simulink model "lab2_teste"  (R2017a)
settings: Solver=ode3  StartTime=0.0  StopTime=10.0  RelTol=1e-3  EnableMultiTasking=on
values from neighbouring files (symbols this model uses):
  input_amplitude = 1    [test2_square_half_hz.mat]
  input_frequency = 0.5    [test2_square_half_hz.mat]
  sampling_time = 0.02    [prbs_good_b0-098.mat]    (also in test2_square_half_hz.mat)
undefined symbols (not defined in the file or in its folder): MIO, National_Instruments, PCI
libraries: sldrtlib x3
settings Model: SimulationMode=external  ExtModeTrigDuration=20000  Creator=alunos  LastModifiedBy=jmgri
settings DataIOCC: SaveFormat=Array
settings DebuggingCC: SFUnexpectedBacktrackingDiag=warning  SFNoUnconditionalDefaultTransitionDiag=warning  SFExecutionAtInitializationDiag=none
settings HardwareCC: TargetIntDivRoundTo=Zero  TargetEndianess=LittleEndian  TargetHWDeviceType=Intel->x86/Pentium
settings ModelReferenceCC: PropagateSignalLabelsOutOfModel=off
settings RTWCC: SystemTargetFile=sldrt.tlc  TemplateMakefile=sldrt.tmf  Description=Simulink Desktop Real-Time  RTWCompilerOptimization=on
settings CodeAppCC: MaxIdLength=95
settings SimulinkDesktopRealTimeCC: TargetPreCompLibLocation=C:\Program Files\MATLAB\R2017a\toolbox\sldrt\lib\win64  TargetLangStandard=C89/C90 (ANSI)  SupportVariableSizeSignals=off
settings ConfigComp: CovMetricSettings=dw  CovHtmlReporting=on  CovSaveCumulativeToWorkspaceVar=on  CovSaveSingleToWorkspaceVar=on  CovExternalEMLEnable=off

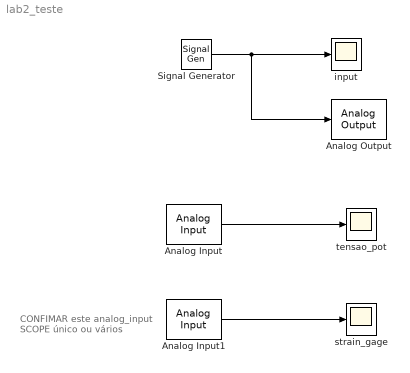
== system lab2_teste ==
  note: CONFIMAR este analog_input
      | SCOPE único ou vários
  Analog Input : sldrtlib/Analog Input  SampleTime=sampling_time  MaxMissedTicks=10  ShowMissedTicks=off  YieldWhenWaiting=off  DrvName=National_Instruments/PCI-MIO-16E-4  DrvAddress=4294967295  DrvOptions=[0 0 0 0 0 0]  Channels=1  RangeMode=1  VoltRange=1  DataType=1
      settings: AttributesFormatString=National Instruments\nPCI-MIO-16E-4 [auto]  SourceProductName=Simulink Desktop Real-Time
  Analog Input1 : sldrtlib/Analog Input  SampleTime=sampling_time  MaxMissedTicks=10  ShowMissedTicks=off  YieldWhenWaiting=off  DrvName=National_Instruments/PCI-MIO-16E-4  DrvAddress=4294967295  DrvOptions=[0 0 0 0 0 0]  Channels=2  RangeMode=1  VoltRange=1  DataType=1
      settings: AttributesFormatString=National Instruments\nPCI-MIO-16E-4 [auto]  SourceProductName=Simulink Desktop Real-Time
  Analog Output : sldrtlib/Analog Output  SampleTime=sampling_time  MaxMissedTicks=10  ShowMissedTicks=off  YieldWhenWaiting=off  DrvName=National_Instruments/PCI-MIO-16E-4  DrvAddress=4294967295  DrvOptions=[0 0 0 0 0 0]  Channels=1  RangeMode=1  VoltRange=1  InitialValue=0  FinalValue=0
      settings: AttributesFormatString=National Instruments\nPCI-MIO-16E-4 [auto]  SourceProductName=Simulink Desktop Real-Time
  Signal Generator : SignalGenerator  WaveForm=square  Amplitude=input_amplitude  Frequency=input_frequency
  input : Scope
  strain_gage : Scope
  tensao_pot : Scope
  wires:
  Signal Generator/1 -> Analog Output/1, input/1
  Analog Input/1 -> tensao_pot/1
  Analog Input1/1 -> strain_gage/1
